simulink model "OMAP"  (R2018b)
settings: Solver=FixedStepDiscrete  StartTime=0.0  StopTime=10.0  FixedStep=0.01  RelTol=1e-3
values from neighbouring files (symbols this model uses):
  Clb_ICADirect_LaneDisp_StateFive = Simulink.Parameter    [omap_ver_442.m]
  Clb_ICADirect_LaneDisp_StateFour = Simulink.Parameter    [omap_ver_442.m]
  Clb_ICADirect_LaneDisp_StateOne = Simulink.Parameter    [omap_ver_442.m]
  Clb_ICADirect_LaneDisp_StateThree = Simulink.Parameter    [omap_ver_442.m]
  Clb_ICADirect_LaneDisp_StateTwo = Simulink.Parameter    [omap_ver_442.m]
  Clb_ICADirect_LaneDisp_StateZero = Simulink.Parameter    [omap_ver_442.m]
  Clb_ICADirect_LaneDispSW = Simulink.Parameter    [omap_ver_442.m]
  Clb_ICADirect_TrnLghtsCom_Switch = Simulink.Parameter    [omap_ver_442.m]
  Clb_ICADirect_TrnLghtsCom_Value = Simulink.Parameter    [omap_ver_442.m]
  Clb_ICADirect_TrnLghtsCrtl_Inhb = Simulink.Parameter    [omap_ver_442.m]
  OMAP_ACCAEB_EMSESC_Decel = Simulink.Parameter    [omap_ver_442.m]
  OMAP_ACCFCW_IC_Decel = Simulink.Parameter    [omap_ver_442.m]
  OMAP_clb_ACC_RVVReqType = Simulink.Parameter    [omap_ver_442.m]
  OMAP_clb_ACC_RVVReqType_Switch = Simulink.Parameter    [omap_ver_442.m]
  OMAP_clb_ACCHeadwayDisplay = Simulink.Parameter    [omap_ver_442.m]
  OMAP_clb_ACCHeadwayDisplay_Switch = Simulink.Parameter    [omap_ver_442.m]
  OMAP_clb_ACCHeadwayIcon = Simulink.Parameter    [omap_ver_442.m]
  OMAP_clb_ACCHeadwayIcon_Switch = Simulink.Parameter    [omap_ver_442.m]
  OMAP_clb_ACCMessagePrompt = Simulink.Parameter    [omap_ver_442.m]
  OMAP_clb_ACCMessagePrompt_Switch = Simulink.Parameter    [omap_ver_442.m]
  OMAP_clb_ACCRequestEPB = Simulink.Parameter    [omap_ver_442.m]
  OMAP_clb_ACCRequestEPB_Switch = Simulink.Parameter    [omap_ver_442.m]
  OMAP_clb_ACCSetSpeed = Simulink.Parameter    [omap_ver_442.m]
  OMAP_clb_ACCSetSpeed_Switch = Simulink.Parameter    [omap_ver_442.m]
  OMAP_clb_ACCSetSpeedDis = Simulink.Parameter    [omap_ver_442.m]
  OMAP_clb_ACCSetSpeedDis_Switch = Simulink.Parameter    [omap_ver_442.m]
  OMAP_clb_ACCState = Simulink.Parameter    [omap_ver_442.m]
  OMAP_clb_ACCState_Switch = Simulink.Parameter    [omap_ver_442.m]
  OMAP_clb_ACCStatusIconDis = Simulink.Parameter    [omap_ver_442.m]
  OMAP_clb_ACCStatusIconDis_Switch = Simulink.Parameter    [omap_ver_442.m]
  OMAP_clb_ACCTorqueReq = Simulink.Parameter    [omap_ver_442.m]
  OMAP_clb_ACCTorqueReq_Switch = Simulink.Parameter    [omap_ver_442.m]
  OMAP_clb_ADAS_State = Simulink.Parameter    [omap_ver_442.m]
  OMAP_clb_ADAS_State_Switch = Simulink.Parameter    [omap_ver_442.m]
  OMAP_clb_AEBAlertReq = Simulink.Parameter    [omap_ver_442.m]
  OMAP_clb_AEBAlertReq_Switch = Simulink.Parameter    [omap_ver_442.m]
  OMAP_clb_AEBBrakingProg = Simulink.Parameter    [omap_ver_442.m]
  OMAP_clb_AEBBrakingProg_Switch = Simulink.Parameter    [omap_ver_442.m]
  OMAP_clb_AEBFaultStatus = Simulink.Parameter    [omap_ver_442.m]
  OMAP_clb_AEBFaultStatus_Switch = Simulink.Parameter    [omap_ver_442.m]
  OMAP_clb_AEBMassageDisp = Simulink.Parameter    [omap_ver_442.m]
  OMAP_clb_AEBMassageDisp_Switch = Simulink.Parameter    [omap_ver_442.m]
  OMAP_clb_AEBState = Simulink.Parameter    [omap_ver_442.m]
  OMAP_clb_AEBState_Switch = Simulink.Parameter    [omap_ver_442.m]
  OMAP_clb_AEBSwitchStatus = Simulink.Parameter    [omap_ver_442.m]
  OMAP_clb_AEBSwitchStatus_Switch = Simulink.Parameter    [omap_ver_442.m]
  OMAP_clb_BrakeRequest = Simulink.Parameter    [omap_ver_442.m]
  OMAP_clb_BrakeRequest_Switch = Simulink.Parameter    [omap_ver_442.m]
  OMAP_clb_DecelerationSet = Simulink.Parameter    [omap_ver_442.m]
  OMAP_clb_DecelerationSet_Switch = Simulink.Parameter    [omap_ver_442.m]
  OMAP_clb_DecelerationType = Simulink.Parameter    [omap_ver_442.m]
  OMAP_clb_DecelerationType_Switch = Simulink.Parameter    [omap_ver_442.m]
  OMAP_clb_DeclControlReq = Simulink.Parameter    [omap_ver_442.m]
  OMAP_clb_DeclControlReq_Switch = Simulink.Parameter    [omap_ver_442.m]
  OMAP_clb_DownorUpGearMinTime = Simulink.Parameter    [omap_ver_442.m]
  OMAP_clb_DownorUpGearMinTime_Switch = Simulink.Parameter    [omap_ver_442.m]
  OMAP_clb_ELKPopupMessage = Simulink.Parameter    [omap_ver_442.m]
  OMAP_clb_ELKPopupMessage_Switch = Simulink.Parameter    [omap_ver_442.m]
  OMAP_clb_ELKSts = Simulink.Parameter    [omap_ver_442.m]
  OMAP_clb_ELKSts_Switch = Simulink.Parameter    [omap_ver_442.m]
  OMAP_clb_ESAFaultSt = Simulink.Parameter    [omap_ver_442.m]
  OMAP_clb_ESAFaultSt_Switch = Simulink.Parameter    [omap_ver_442.m]
  OMAP_clb_ESARequest = Simulink.Parameter    [omap_ver_442.m]
  OMAP_clb_ESARequest_Switch = Simulink.Parameter    [omap_ver_442.m]
  OMAP_clb_ESAState = Simulink.Parameter    [omap_ver_442.m]
  OMAP_clb_ESAState_Switch = Simulink.Parameter    [omap_ver_442.m]
  OMAP_clb_ESATorqueReq = Simulink.Parameter    [omap_ver_442.m]
  OMAP_clb_ESATorqueReq_Switch = Simulink.Parameter    [omap_ver_442.m]
  OMAP_clb_ESCDriveOff = Simulink.Parameter    [omap_ver_442.m]
  OMAP_clb_ESCDriveOff_Switch = Simulink.Parameter    [omap_ver_442.m]
  OMAP_clb_ESCHoldReq = Simulink.Parameter    [omap_ver_442.m]
  OMAP_clb_ESCHoldReq_Switch = Simulink.Parameter    [omap_ver_442.m]
  OMAP_clb_Handsoffwarning = Simulink.Parameter    [omap_ver_442.m]
  OMAP_clb_Handsoffwarning_Switch = Simulink.Parameter    [omap_ver_442.m]
  OMAP_clb_HapticAlarmReq = Simulink.Parameter    [omap_ver_442.m]
  OMAP_clb_HapticAlarmReq_Switch = Simulink.Parameter    [omap_ver_442.m]
  OMAP_clb_HMIPopupMassage = Simulink.Parameter    [omap_ver_442.m]
  OMAP_clb_HMIPopupMassage_Switch = Simulink.Parameter    [omap_ver_442.m]
  OMAP_clb_HWAActionSts = Simulink.Parameter    [omap_ver_442.m]
  OMAP_clb_HWAActionSts_Switch = Simulink.Parameter    [omap_ver_442.m]
  OMAP_clb_HWAMode = Simulink.Parameter    [omap_ver_442.m]
  OMAP_clb_HWAMode_Switch = Simulink.Parameter    [omap_ver_442.m]
  OMAP_clb_HWATurnOnIdctr = Simulink.Parameter    [omap_ver_442.m]
  OMAP_clb_HWATurnOnIdctr_Switch = Simulink.Parameter    [omap_ver_442.m]
  OMAP_clb_ICAMassageDisp = Simulink.Parameter    [omap_ver_442.m]
  OMAP_clb_ICAMassageDisp_Switch = Simulink.Parameter    [omap_ver_442.m]
  OMAP_clb_ICAStatusIcon = Simulink.Parameter    [omap_ver_442.m]
  OMAP_clb_ICAStatusIcon_Switch = Simulink.Parameter    [omap_ver_442.m]
  OMAP_clb_ISLCDriverRemind = Simulink.Parameter    [omap_ver_442.m]
  OMAP_clb_ISLCDriverRemind_Switch = Simulink.Parameter    [omap_ver_442.m]
  OMAP_clb_ISLCState = Simulink.Parameter    [omap_ver_442.m]
  OMAP_clb_ISLCState_Switch = Simulink.Parameter    [omap_ver_442.m]
  OMAP_clb_JAFaultSt = Simulink.Parameter    [omap_ver_442.m]
  OMAP_clb_JAFaultSt_Switch = Simulink.Parameter    [omap_ver_442.m]
  OMAP_clb_LCAPopupMessage = Simulink.Parameter    [omap_ver_442.m]
  OMAP_clb_LCAPopupMessage_Switch = Simulink.Parameter    [omap_ver_442.m]
  OMAP_clb_LCAStatusDisplay = Simulink.Parameter    [omap_ver_442.m]
  OMAP_clb_LCAStatusDisplay_Switch = Simulink.Parameter    [omap_ver_442.m]
  OMAP_clb_LDWStatusDisplay = Simulink.Parameter    [omap_ver_442.m]
  OMAP_clb_LDWStatusDisplay_Switch = Simulink.Parameter    [omap_ver_442.m]
  OMAP_clb_LDWWarningSt = Simulink.Parameter    [omap_ver_442.m]
  OMAP_clb_LDWWarningSt_Switch = Simulink.Parameter    [omap_ver_442.m]
  OMAP_clb_LightControlValid = Simulink.Parameter    [omap_ver_442.m]
  OMAP_clb_LightControlValid_Switch = Simulink.Parameter    [omap_ver_442.m]
  OMAP_clb_LKAActivation = Simulink.Parameter    [omap_ver_442.m]
  OMAP_clb_LKAActivation_Switch = Simulink.Parameter    [omap_ver_442.m]
  OMAP_clb_LKAAngleReq = Simulink.Parameter    [omap_ver_442.m]
  OMAP_clb_LKAAngleReq_Switch = Simulink.Parameter    [omap_ver_442.m]
  OMAP_clb_LKAMode = Simulink.Parameter    [omap_ver_442.m]
  OMAP_clb_LKAMode_Switch = Simulink.Parameter    [omap_ver_442.m]
  OMAP_clb_LKAorELK_CoolTime = Simulink.Parameter    [omap_ver_442.m]
  OMAP_clb_LKAState = Simulink.Parameter    [omap_ver_442.m]
  OMAP_clb_LKAState_Switch = Simulink.Parameter    [omap_ver_442.m]
  OMAP_clb_LKAStatusDisplay = Simulink.Parameter    [omap_ver_442.m]
  OMAP_clb_LKAStatusDisplay_Switch = Simulink.Parameter    [omap_ver_442.m]
  OMAP_clb_LKASwitchState = Simulink.Parameter    [omap_ver_442.m]
  OMAP_clb_LKASwitchState_Switch = Simulink.Parameter    [omap_ver_442.m]
  OMAP_clb_LKATorqFactReq = Simulink.Parameter    [omap_ver_442.m]
  OMAP_clb_LKATorqFactReq_Switch = Simulink.Parameter    [omap_ver_442.m]
  OMAP_clb_PrefillRequest = Simulink.Parameter    [omap_ver_442.m]
  ... (+36 more)
libraries: simulink x184, canmsglib x2
(part 5 of 14)

== system OMAP/Runnable_OMAP_10ms_sys/OMAP_Module/Default_IC ==
  Bus Creator16 : BusCreator  Inputs=36
  Constant3 : Constant  Value=0  OutDataTypeStr=uint8
  Constant4 : Constant  Value=0  OutDataTypeStr=uint8
  OMAPve_y_ACC_DesiredHeadway_DisplayNum : Constant  Value=0  OutDataTypeStr=uint8
  OMAPve_y_ACC_DesiredHeadway_Icon_BasicNum : Constant  Value=0  OutDataTypeStr=uint8
  OMAPve_y_ACC_Desired_Set_SpeedNum : Constant  Value=0  OutDataTypeStr=uint8
  OMAPve_y_ACC_HMI_TgtDisp_FlagNum : Constant  Value=0  OutDataTypeStr=uint8
  OMAPve_y_ACC_Pop_Up_MessageNum : Constant  Value=0  OutDataTypeStr=uint8
  OMAPve_y_ACC_Set_Speed_DisplayNum : Constant  Value=0  OutDataTypeStr=uint8
  OMAPve_y_ACC_Vehicle_Icon_DisplayNum : Constant  Value=0  OutDataTypeStr=uint8
  OMAPve_y_ADAS_ELKStsNum1 : Constant  Value=0  OutDataTypeStr=uint8
  OMAPve_y_ADAS_HWAActionSts : Constant  Value=0  OutDataTypeStr=uint8
  OMAPve_y_ADAS_HWAMode : Constant  Value=0  OutDataTypeStr=uint8
  OMAPve_y_ADAS_HWATurnOnIndicator : Constant  Value=0  OutDataTypeStr=uint8
  OMAPve_y_ADAS_ISLCDriverRemind1 : Constant  Value=0  OutDataTypeStr=uint8
  OMAPve_y_ADAS_ISLCState1 : Constant  Value=0  OutDataTypeStr=uint8
  OMAPve_y_ADAS_JAFaultSt_2 : Constant  Value=0  OutDataTypeStr=uint8
  OMAPve_y_ADAS_LightControlValid : Constant  Value=0  OutDataTypeStr=uint8
  OMAPve_y_ADAS_TurnLightsCommand1 : Constant  Value=0  OutDataTypeStr=uint8
  OMAPve_y_AEB_Alert_ReqNum : Constant  Value=0  OutDataTypeStr=uint8
  OMAPve_y_AEB_Fault_StatusNum : Constant  Value=0  OutDataTypeStr=uint8
  OMAPve_y_AEB_Switch_StatusNum : Constant  Value=0  OutDataTypeStr=uint8
  OMAPve_y_AEB_tipsNum : Constant  Value=0  OutDataTypeStr=uint8
  OMAPve_y_HMI_Popup_StatusNum : Constant  Value=0  OutDataTypeStr=uint8
  OMAPve_y_Hands_off_warningNum : Constant  Value=0  OutDataTypeStr=uint8
  OMAPve_y_ICA_HMI_Txt_DispNum : Constant  Value=0  OutDataTypeStr=uint8
  OMAPve_y_LDW_FlagNum : Constant  Value=0  OutDataTypeStr=uint8
  OMAPve_y_LDW_Status_DisplayNum : Constant  Value=0  OutDataTypeStr=uint8
  OMAPve_y_LKA_Mode_from_CameraNum : Constant  Value=0  OutDataTypeStr=uint8
  OMAPve_y_LKA_Status_DisplayNum : Constant  Value=0  OutDataTypeStr=uint8
  OMAPve_y_LKA_Switch_StateNum : Constant  Value=0  OutDataTypeStr=uint8
  OMAPve_y_LKA_action_indicationNum : Constant  Value=0  OutDataTypeStr=uint8
  OMAPve_y_RVVACC_Vehiclespeed_request_typeNum : Constant  Value=0  OutDataTypeStr=uint8
  OMAPve_y_TARGET_POSITIONNum : Constant  Value=0  OutDataTypeStr=uint8
  OMAPve_y_TJA_status_iconNum : Constant  Value=0  OutDataTypeStr=uint8
  OMAPve_y_TSR_Vision_Only_Sign_TypeNum : Constant  Value=0  OutDataTypeStr=uint8
  OMAPve_y_Vehicle_Lane_DisplayNum : Constant  Value=0  OutDataTypeStr=uint8
  Default_IC : Outport
  wires:
  OMAPve_y_LKA_Status_DisplayNum/1 -> Bus Creator16/31  "OMAPve_y_LKA_Status_Display_2"
  OMAPve_y_ACC_Desired_Set_SpeedNum/1 -> Bus Creator16/11  "OMAPve_y_ACC_Desired_Set_Speed_2"
  OMAPve_y_AEB_tipsNum/1 -> Bus Creator16/19  "OMAPve_y_AEB_tips_2"
  OMAPve_y_ACC_Pop_Up_MessageNum/1 -> Bus Creator16/15  "OMAPve_y_ACC_Pop_Up_Message_2"
  OMAPve_y_LDW_Status_DisplayNum/1 -> Bus Creator16/29  "OMAPve_y_LDW_Status_Display_2"
  OMAPve_y_AEB_Switch_StatusNum/1 -> Bus Creator16/18  "OMAPve_y_AEB_Switch_Status_2"
  OMAPve_y_ACC_DesiredHeadway_Icon_BasicNum/1 -> Bus Creator16/10  "OMAPve_y_ACC_DesiredHeadway_Icon_Basic_2"
  OMAPve_y_ICA_HMI_Txt_DispNum/1 -> Bus Creator16/35  "OMAPve_y_ICA_HMI_Txt_Disp_2"
  OMAPve_y_TARGET_POSITIONNum/1 -> Bus Creator16/22  "OMAPve_y_TARGET_POSITION_2"
  OMAPve_y_ACC_Vehicle_Icon_DisplayNum/1 -> Bus Creator16/13  "OMAPve_y_ACC_Vehicle_Icon_Display_2"
  OMAPve_y_ACC_DesiredHeadway_DisplayNum/1 -> Bus Creator16/9  "OMAPve_y_ACC_DesiredHeadway_Display_2"
  OMAPve_y_AEB_Alert_ReqNum/1 -> Bus Creator16/16  "OMAPve_y_AEB_Alert_Req_2"
  OMAPve_y_ACC_Set_Speed_DisplayNum/1 -> Bus Creator16/12  "OMAPve_y_ACC_Set_Speed_Display_2"
  OMAPve_y_LKA_action_indicationNum/1 -> Bus Creator16/33  "OMAPve_y_LKA_action_indication_2"
  OMAPve_y_Hands_off_warningNum/1 -> Bus Creator16/25  "OMAPve_y_Hands_off_warning_2"
  OMAPve_y_RVVACC_Vehiclespeed_request_typeNum/1 -> Bus Creator16/14  "OMAPve_y_RVVACC_Vehiclespeed_request_type_2"
  OMAPve_y_LKA_Mode_from_CameraNum/1 -> Bus Creator16/30  "OMAPve_y_LKA_Mode_from_Camera_2"
  OMAPve_y_ACC_HMI_TgtDisp_FlagNum/1 -> Bus Creator16/21  "OMAPve_y_ACC_HMI_TgtDisp_Flag_2"
  OMAPve_y_HMI_Popup_StatusNum/1 -> Bus Creator16/26  "OMAPve_y_HMI_Popup_Status_2"
  OMAPve_y_TSR_Vision_Only_Sign_TypeNum/1 -> Bus Creator16/8  "OMAPve_y_TSR_Vision_Only_Sign_Type_2"
  OMAPve_y_TJA_status_iconNum/1 -> Bus Creator16/36  "OMAPve_y_TJA_status_icon_2"
  OMAPve_y_AEB_Fault_StatusNum/1 -> Bus Creator16/17  "OMAPve_y_AEB_Fault_Status_2"
  OMAPve_y_Vehicle_Lane_DisplayNum/1 -> Bus Creator16/27  "OMAPve_y_Vehicle_Lane_Display_2"
  OMAPve_y_LKA_Switch_StateNum/1 -> Bus Creator16/32  "OMAPve_y_LKA_Switch_State_2"
  OMAPve_y_LDW_FlagNum/1 -> Bus Creator16/28  "OMAPve_y_LDW_Flag_2"
  Bus Creator16/1 -> Default_IC/1  "Default_IC"
  OMAPve_y_ADAS_ELKStsNum1/1 -> Bus Creator16/34  "OMAPve_y_ADAS_ELKSts_2"
  OMAPve_y_ADAS_JAFaultSt_2/1 -> Bus Creator16/20  "OMAPve_y_ADAS_JAFaultSt_2"
  OMAPve_y_ADAS_ISLCState1/1 -> Bus Creator16/23  "OMAPve_y_ADAS_ISLCState_2"
  OMAPve_y_ADAS_ISLCDriverRemind1/1 -> Bus Creator16/24  "OMAPve_y_ADAS_ISLCDriverRemind_2"
  OMAPve_y_ADAS_LightControlValid/1 -> Bus Creator16/6  "OMAPve_y_ADAS_LightControlValid_2"
  OMAPve_y_ADAS_HWAActionSts/1 -> Bus Creator16/4  "OMAPve_y_ADAS_HWAActionSts_2"
  OMAPve_y_ADAS_HWATurnOnIndicator/1 -> Bus Creator16/3  "OMAPve_y_ADAS_HWATurnOnIndicator_2"
  OMAPve_y_ADAS_HWAMode/1 -> Bus Creator16/7  "OMAPve_y_ADAS_HWAMode_2"
  OMAPve_y_ADAS_TurnLightsCommand1/1 -> Bus Creator16/5  "OMAPve_y_ADAS_TurnLightsCommand_2"
  Constant3/1 -> Bus Creator16/2  "OMAPve_y_ADAS_ESAFaultSt_2"
  Constant4/1 -> Bus Creator16/1  "OMAPve_y_ADAS_ELKPopupMessage_2"

== system OMAP/Runnable_OMAP_10ms_sys/OMAP_Module/Default_OTHER ==
  Bus Creator26 : BusCreator  Inputs=5
  Data Type Conversion72 : DataTypeConversion  OutDataTypeStr=uint8
  Delay : Delay
  NOT : Logic  Operator=NOT  IconShape=distinctive  AllPortsSameDT=off  OutDataTypeStr=boolean
  OMAPve_y_ABS_ESP_power_cut_request2Num1 : Constant  Value=0  OutDataTypeStr=uint8
  OMAPve_y_ASR_connection_dis_demand2Num1 : Constant  Value=0  OutDataTypeStr=uint8
  OMAPve_y_ECU_operating_phaseNum1 : Constant  Value=9  OutDataTypeStr=uint8
  OMAPve_y_Radar_StateNum1 : Constant  Value=2  OutDataTypeStr=uint8
  Default : Outport
  wires:
  OMAPve_y_ASR_connection_dis_demand2Num1/1 -> Bus Creator26/2  "OMAPve_y_ASR_connection_dis_demand2_2"
  OMAPve_y_ABS_ESP_power_cut_request2Num1/1 -> Bus Creator26/1  "OMAPve_y_ABS_ESP_power_cut_request2_2"
  Data Type Conversion72/1 -> Bus Creator26/3  "OMAPve_y_TYPE_RAPPORT_2"
  Bus Creator26/1 -> Default/1  "Default"
  OMAPve_y_Radar_StateNum1/1 -> Bus Creator26/5  "OMAPve_y_Radar_State_2"
  OMAPve_y_ECU_operating_phaseNum1/1 -> Bus Creator26/4  "OMAPve_y_ECU_operating_phase_2"
  NOT/1 -> Delay/1, Data Type Conversion72/1
  Delay/1 -> NOT/1

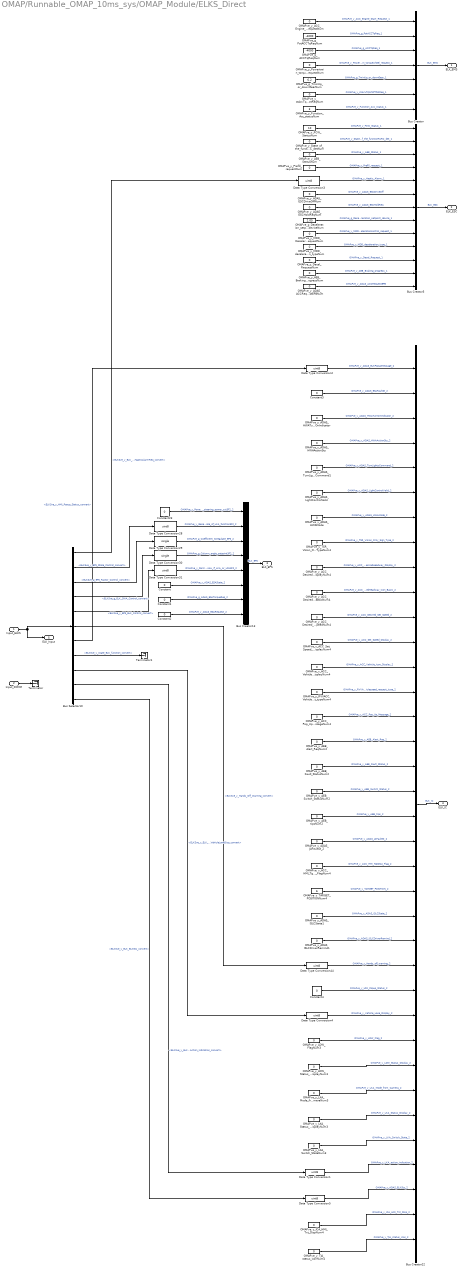
== system OMAP/Runnable_OMAP_10ms_sys/OMAP_Module/ELKS_Direct ==
  Input_ELKS : Inport
  Input_FDMM : Inport  Port=2
  Bus Creator : BusCreator  Inputs=7
  Bus Creator13 : BusCreator  Inputs=8
  Bus Creator22 : BusCreator  Inputs=36
  Bus Creator5 : BusCreator  Inputs=13
  Bus Selector10 : BusSelector  OutputSignals=ELKSve_y_ELK_HapticAlarmReq_convert,ELKSve_y_EPS_State_Control_convert,ELKSve_g_EPS_Factor_Control_convert,ELKSve_g_ELK_SWA_Control_convert,ELKSve_y_EPS_ELK_Control_convert,ELKSve_y_Hands_Off_Warning_convert,ELKSve_y_HMI_Popup_Status_convert,ELKSve_y_state_ELK_function_convert,ELKSve_y_ELK_VehicleLaneDisp_convert,ELKSve_y_ELK_Action_Indication_convert,ELKSve_y_ELK_ELKSts_convert
  Constant{,2..4,23} (5 alike) : Constant  Value=0  OutDataTypeStr=uint8
  Constant1 : Constant  Value=0  OutDataTypeStr=single
  Data Type Conversion{1..5,28,31,44} (8 alike) : DataTypeConversion  OutDataTypeStr=uint8
  Data Type Conversion29 : DataTypeConversion  OutDataTypeStr=single
  Data Type Conversion30 : DataTypeConversion  OutDataTypeStr=single
  OMAPve_g_ACCTqReqNum : Constant  Value=-4000  OutDataTypeStr=single
  OMAPve_g_Deceleration_setpoint_deviceNum : Constant  Value=2.05  OutDataTypeStr=single
  OMAPve_g_PotACCTqReqNum : Constant  Value=-4000  OutDataTypeStr=single
  OMAPve_g_TminUp_or_downGearNum : Constant  Value=6.2  OutDataTypeStr=single
  OMAPve_y_ACC_DesiredHeadway_DisplayNum4 : Constant  Value=0  OutDataTypeStr=uint8
  OMAPve_y_ACC_DesiredHeadway_Icon_BasicNum4 : Constant  Value=0  OutDataTypeStr=uint8
  OMAPve_y_ACC_Desired_Set_SpeedNum4 : Constant  Value=0  OutDataTypeStr=uint8
  OMAPve_y_ACC_Engine_Start_RequestNum : Constant  Value=0  OutDataTypeStr=uint8
  OMAPve_y_ACC_HMI_TgtDisp_FlagNum4 : Constant  Value=0  OutDataTypeStr=uint8
  OMAPve_y_ACC_Pop_Up_MessageNum4 : Constant  Value=0  OutDataTypeStr=uint8
  OMAPve_y_ACC_Set_Speed_DisplayNum4 : Constant  Value=0  OutDataTypeStr=uint8
  OMAPve_y_ACC_Vehicle_Icon_DisplayNum4 : Constant  Value=0  OutDataTypeStr=uint8
  OMAPve_y_ADAS_ACCRequestEPBNum : Constant  Value=0  OutDataTypeStr=uint8
  OMAPve_y_ADAS_ESCDriveOffNum : Constant  Value=0  OutDataTypeStr=uint8
  OMAPve_y_ADAS_ESCHoldReqNum : Constant  Value=0  OutDataTypeStr=uint8
  OMAPve_y_ADAS_HWAActionSts : Constant  Value=0  OutDataTypeStr=uint8
  OMAPve_y_ADAS_HWAMode : Constant  Value=0  OutDataTypeStr=uint8
  OMAPve_y_ADAS_HWATurnOnIndicator : Constant  Value=0  OutDataTypeStr=uint8
  OMAPve_y_ADAS_ISLCDriverRemind1 : Constant  Value=0  OutDataTypeStr=uint8
  OMAPve_y_ADAS_ISLCState1 : Constant  Value=0  OutDataTypeStr=uint8
  OMAPve_y_ADAS_JAFaultSt_2 : Constant  Value=0  OutDataTypeStr=uint8
  OMAPve_y_ADAS_LightControlValid : Constant  Value=0  OutDataTypeStr=uint8
  OMAPve_y_ADAS_TurnLightsCommand1 : Constant  Value=0  OutDataTypeStr=uint8
  OMAPve_y_AEB_Alert_ReqNum2 : Constant  Value=0  OutDataTypeStr=uint8
  OMAPve_y_AEB_Braking_progressNum : Constant  Value=0  OutDataTypeStr=uint8
  OMAPve_y_AEB_Fault_StatusNum2 : Constant  Value=0  OutDataTypeStr=uint8
  OMAPve_y_AEB_StatusNum : Constant  Value=0  OutDataTypeStr=uint8
  OMAPve_y_AEB_Switch_StatusNum2 : Constant  Value=0  OutDataTypeStr=uint8
  OMAPve_y_AEB_tipsNum2 : Constant  Value=0  OutDataTypeStr=uint8
  OMAPve_y_Decel_RequestNum : Constant  Value=0  OutDataTypeStr=uint8
  OMAPve_y_FCW_StatusNum : Constant  Value=10  OutDataTypeStr=uint8
  OMAPve_y_Function_Acc_statusNum : Constant  Value=3  OutDataTypeStr=uint8
  OMAPve_y_ICA_HMI_Txt_DispNum4 : Constant  Value=0  OutDataTypeStr=uint8
  OMAPve_y_LDW_FlagNum3 : Constant  Value=0  OutDataTypeStr=uint8
  OMAPve_y_LDW_Status_DisplayNum3 : Constant  Value=0  OutDataTypeStr=uint8
  OMAPve_y_LKA_Mode_from_CameraNum3 : Constant  Value=0  OutDataTypeStr=uint8
  OMAPve_y_LKA_Status_DisplayNum3 : Constant  Value=0  OutDataTypeStr=uint8
  OMAPve_y_LKA_Switch_StateNum3 : Constant  Value=0  OutDataTypeStr=uint8
  OMAPve_y_MDD_Decelerationcontrol_requestNum : Constant  Value=0  OutDataTypeStr=uint8
  OMAPve_y_MDD_deceleration_typeNum : Constant  Value=0  OutDataTypeStr=uint8
  OMAPve_y_Powertrain_torquewheel_requestNum : Constant  Value=0  OutDataTypeStr=uint8
  OMAPve_y_Prefill_requestNum : Constant  Value=0  OutDataTypeStr=uint8
  OMAPve_y_RVVACC_Vehiclespeed_request_typeNum4 : Constant  Value=0  OutDataTypeStr=uint8
  OMAPve_y_State_of_the_functionFARC_detNum : Constant  Value=0  OutDataTypeStr=uint8
  OMAPve_y_TARGET_POSITIONNum4 : Constant  Value=6  OutDataTypeStr=uint8
  OMAPve_y_TJA_status_iconNum4 : Constant  Value=0  OutDataTypeStr=uint8
  OMAPve_y_TSR_Vision_Only_Sign_TypeNum4 : Constant  Value=0  OutDataTypeStr=uint8
  OMAPve_y_stAcvTqWhlPTPotReqNum : Constant  Value=0  OutDataTypeStr=uint8
  Terminator : Terminator
  Terminator1 : Terminator
  ELK_EMS : Outport
  ELK_ESC : Outport  Port=2
  ELK_EPS : Outport  Port=3
  ELK_IC : Outport  Port=4
  ELK_Input : Outport  Port=5
  wires:
  Bus Creator22/1 -> ELK_IC/1  "ELK_IC"
  Data Type Conversion44/1 -> Bus Creator22/25  "OMAPve_y_Hands_off_warning_2"
  Data Type Conversion1/1 -> Bus Creator22/33  "OMAPve_y_LKA_action_indication_2"
  Bus Selector10/5 -> Data Type Conversion31/1  "<ELKSve_y_EPS_ELK_Control_convert>"
  Bus Selector10/2 -> Data Type Conversion28/1  "<ELKSve_y_EPS_State_Control_convert>"
  Data Type Conversion29/1 -> Bus Creator13/3  "OMAPve_g_Coefficient_toregulate_EPS_2"
  OMAPve_y_LDW_Status_DisplayNum3/1 -> Bus Creator22/29  "OMAPve_y_LDW_Status_Display_2"
  OMAPve_y_LDW_FlagNum3/1 -> Bus Creator22/28  "OMAPve_y_LDW_Flag_2"
  OMAPve_y_ACC_DesiredHeadway_Icon_BasicNum4/1 -> Bus Creator22/10  "OMAPve_y_ACC_DesiredHeadway_Icon_Basic_2"
  Bus Selector10/6 -> Data Type Conversion44/1  "<ELKSve_y_Hands_Off_Warning_convert>"
  Bus Selector10/4 -> Data Type Conversion30/1  "<ELKSve_g_ELK_SWA_Control_convert>"
  OMAPve_y_ACC_HMI_TgtDisp_FlagNum4/1 -> Bus Creator22/21  "OMAPve_y_ACC_HMI_TgtDisp_Flag_2"
  Bus Selector10/3 -> Data Type Conversion29/1  "<ELKSve_g_EPS_Factor_Control_convert>"
  Data Type Conversion4/1 -> Bus Creator22/27  "OMAPve_y_Vehicle_Lane_Display_2"
  OMAPve_y_TJA_status_iconNum4/1 -> Bus Creator22/36  "OMAPve_y_TJA_status_icon_2"
  Bus Selector10/8 -> Terminator1/1  "<ELKSve_y_state_ELK_function_convert>"
  OMAPve_y_TARGET_POSITIONNum4/1 -> Bus Creator22/22  "OMAPve_y_TARGET_POSITION_2"
  OMAPve_y_ACC_Vehicle_Icon_DisplayNum4/1 -> Bus Creator22/13  "OMAPve_y_ACC_Vehicle_Icon_Display_2"
  OMAPve_y_ACC_DesiredHeadway_DisplayNum4/1 -> Bus Creator22/9  "OMAPve_y_ACC_DesiredHeadway_Display_2"
  OMAPve_y_LKA_Status_DisplayNum3/1 -> Bus Creator22/31  "OMAPve_y_LKA_Status_Display_2"
  OMAPve_y_AEB_tipsNum2/1 -> Bus Creator22/19  "OMAPve_y_AEB_tips_2"
  OMAPve_y_ACC_Pop_Up_MessageNum4/1 -> Bus Creator22/15  "OMAPve_y_ACC_Pop_Up_Message_2"
  Bus Selector10/7 -> Data Type Conversion2/1  "<ELKSve_y_HMI_Popup_Status_convert>"
  OMAPve_y_ACC_Desired_Set_SpeedNum4/1 -> Bus Creator22/11  "OMAPve_y_ACC_Desired_Set_Speed_2"
  OMAPve_y_ICA_HMI_Txt_DispNum4/1 -> Bus Creator22/35  "OMAPve_y_ICA_HMI_Txt_Disp_2"
  Bus Creator13/1 -> ELK_EPS/1  "ELK_EPS"
  OMAPve_y_AEB_Fault_StatusNum2/1 -> Bus Creator22/17  "OMAPve_y_AEB_Fault_Status_2"
  Constant4/1 -> Bus Creator22/26  "OMAPve_y_HMI_Popup_Status_2"
  OMAPve_y_AEB_Switch_StatusNum2/1 -> Bus Creator22/18  "OMAPve_y_AEB_Switch_Status_2"
  OMAPve_y_LKA_Mode_from_CameraNum3/1 -> Bus Creator22/30  "OMAPve_y_LKA_Mode_from_Camera_2"
  OMAPve_y_AEB_Alert_ReqNum2/1 -> Bus Creator22/16  "OMAPve_y_AEB_Alert_Req_2"
  OMAPve_y_ACC_Set_Speed_DisplayNum4/1 -> Bus Creator22/12  "OMAPve_y_ACC_Set_Speed_Display_2"
  Input_ELKS/1 -> ELK_Input/1, Bus Selector10/1
  Constant23/1 -> Bus Creator13/1  "OMAPve_y_Power_steering_power_cut3F2_2"
  Data Type Conversion30/1 -> Bus Creator13/4  "OMAPve_g_Column_angle_setpoint3F2_2"
  OMAPve_y_LKA_Switch_StateNum3/1 -> Bus Creator22/32  "OMAPve_y_LKA_Switch_State_2"
  Data Type Conversion28/1 -> Bus Creator13/2  "OMAPve_y_General_state_of_LKA_function3F2_2"
  Data Type Conversion31/1 -> Bus Creator13/5  "OMAPve_y_Permit_to_know_if_LKA_or_LPA3F2_2"
  OMAPve_y_RVVACC_Vehiclespeed_request_typeNum4/1 -> Bus Creator22/14  "OMAPve_y_RVVACC_Vehiclespeed_request_type_2"
  OMAPve_y_TSR_Vision_Only_Sign_TypeNum4/1 -> Bus Creator22/8  "OMAPve_y_TSR_Vision_Only_Sign_Type_2"
  OMAPve_y_Function_Acc_statusNum/1 -> Bus Creator/7  "OMAPve_y_Function_Acc_status_1"
  OMAPve_y_stAcvTqWhlPTPotReqNum/1 -> Bus Creator/6  "OMAPve_y_stAcvTqWhlPTPotReq_1"
  Bus Creator/1 -> ELK_EMS/1  "ELK_EMS"
  OMAPve_y_ACC_Engine_Start_RequestNum/1 -> Bus Creator/1  "OMAPve_y_ACC_Engine_Start_Request_1"
  OMAPve_g_TminUp_or_downGearNum/1 -> Bus Creator/5  "OMAPve_g_TminUp_or_downGear_1"
  OMAPve_g_PotACCTqReqNum/1 -> Bus Creator/2  "OMAPve_g_PotACCTqReq_1"
  OMAPve_y_Powertrain_torquewheel_requestNum/1 -> Bus Creator/4  "OMAPve_y_Powertrain_torquewheel_request_1"
  OMAPve_g_ACCTqReqNum/1 -> Bus Creator/3  "OMAPve_g_ACCTqReq_1"
  OMAPve_g_Deceleration_setpoint_deviceNum/1 -> Bus Creator5/8  "OMAPve_g_Deceleration_setpoint_device_1"
  OMAPve_y_AEB_StatusNum/1 -> Bus Creator5/3  "OMAPve_y_AEB_Status_1"
  Data Type Conversion3/1 -> Bus Creator5/5  "OMAPve_y_Haptic_Alarm_1"
  OMAPve_y_AEB_Braking_progressNum/1 -> Bus Creator5/12  "OMAPve_y_AEB_Braking_progress_1"
  OMAPve_y_FCW_StatusNum/1 -> Bus Creator5/1  "OMAPve_y_FCW_Status_1"
  OMAPve_y_Decel_RequestNum/1 -> Bus Creator5/11  "OMAPve_y_Decel_Request_1"
  OMAPve_y_MDD_Decelerationcontrol_requestNum/1 -> Bus Creator5/9  "OMAPve_y_MDD_Decelerationcontrol_request_1"
  OMAPve_y_MDD_deceleration_typeNum/1 -> Bus Creator5/10  "OMAPve_y_MDD_deceleration_type_1"
  OMAPve_y_State_of_the_functionFARC_detNum/1 -> Bus Creator5/2  "OMAPve_y_State_of_the_functionFARC_det_1"
  OMAPve_y_Prefill_requestNum/1 -> Bus Creator5/4  "OMAPve_y_Prefill_request_1"
  Bus Creator5/1 -> ELK_ESC/1  "ELK_ESC"
  Input_FDMM/1 -> Terminator/1
  Bus Selector10/10 -> Data Type Conversion1/1  "<ELKSve_y_ELK_Action_Indication_convert>"
  Bus Selector10/1 -> Data Type Conversion3/1  "<ELKSve_y_ELK_HapticAlarmReq_convert>"
  Bus Selector10/11 -> Data Type Conversion5/1  "<ELKSve_y_ELK_ELKSts_convert>"
  Bus Selector10/9 -> Data Type Conversion4/1  "<ELKSve_y_ELK_VehicleLaneDisp_convert>"
  Data Type Conversion5/1 -> Bus Creator22/34  "OMAPve_y_ADAS_ELKSts_2"
  OMAPve_y_ADAS_ESCHoldReqNum/1 -> Bus Creator5/7  "OMAPve_y_ADAS_ESCHoldReq"
  OMAPve_y_ADAS_ESCDriveOffNum/1 -> Bus Creator5/6  "OMAPve_y_ADAS_ESCDriveOff"
  OMAPve_y_ADAS_ACCRequestEPBNum/1 -> Bus Creator5/13  "OMAPve_y_ADAS_ACCRequestEPB"
  OMAPve_y_ADAS_JAFaultSt_2/1 -> Bus Creator22/20  "OMAPve_y_ADAS_JAFaultSt_2"
  OMAPve_y_ADAS_ISLCState1/1 -> Bus Creator22/23  "OMAPve_y_ADAS_ISLCState_2"
  OMAPve_y_ADAS_ISLCDriverRemind1/1 -> Bus Creator22/24  "OMAPve_y_ADAS_ISLCDriverRemind_2"
  OMAPve_y_ADAS_LightControlValid/1 -> Bus Creator22/6  "OMAPve_y_ADAS_LightControlValid_2"
  OMAPve_y_ADAS_HWAActionSts/1 -> Bus Creator22/4  "OMAPve_y_ADAS_HWAActionSts_2"
  OMAPve_y_ADAS_HWATurnOnIndicator/1 -> Bus Creator22/3  "OMAPve_y_ADAS_HWATurnOnIndicator_2"
  OMAPve_y_ADAS_HWAMode/1 -> Bus Creator22/7  "OMAPve_y_ADAS_HWAMode_2"
  OMAPve_y_ADAS_TurnLightsCommand1/1 -> Bus Creator22/5  "OMAPve_y_ADAS_TurnLightsCommand_2"
  Constant1/1 -> Bus Creator13/7  "OMAPve_g_ADAS_ESATorqueReq_2"
  Constant/1 -> Bus Creator13/6  "OMAPve_y_ADAS_ESAState_2"
  Constant2/1 -> Bus Creator13/8  "OMAPve_y_ADAS_ESARequest_2"
  Constant3/1 -> Bus Creator22/2  "OMAPve_y_ADAS_ESAFaultSt_2"
  Data Type Conversion2/1 -> Bus Creator22/1  "OMAPve_y_ADAS_ELKPopupMessage_2"

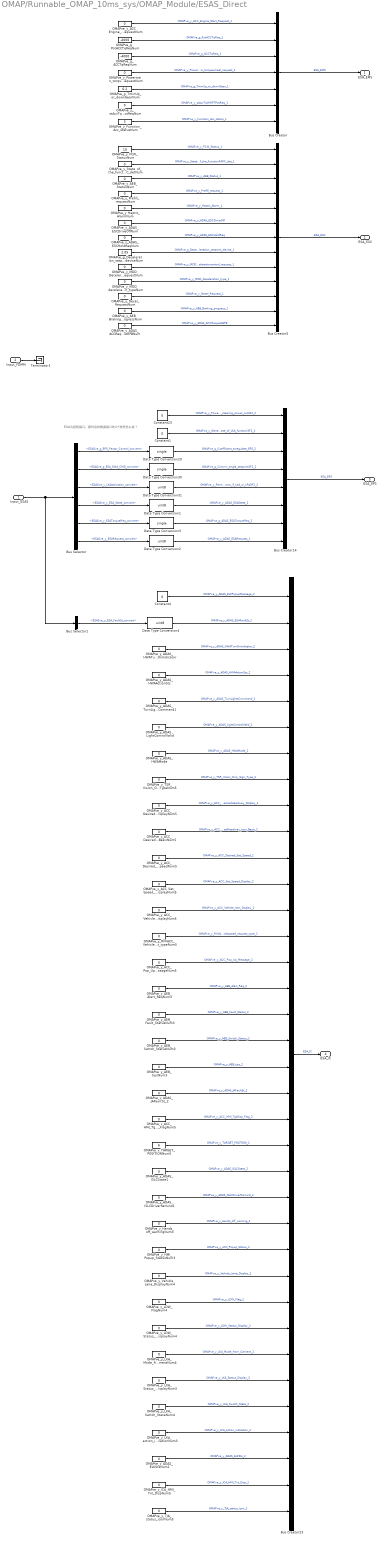
== system OMAP/Runnable_OMAP_10ms_sys/OMAP_Module/ESAS_Direct ==
  note: ESA为扭矩接口。那对应的角度接口的4个信号怎么发？
  Input_ESAS : Inport
  Input_FDMM : Inport  Port=2
  Bus Creator : BusCreator  Inputs=7
  Bus Creator14 : BusCreator  Inputs=8
  Bus Creator23 : BusCreator  Inputs=36
  Bus Creator5 : BusCreator  Inputs=13
  Bus Selector : BusSelector  OutputSignals=ESASve_g_EPS_Factor_Control_convert,ESASve_g_ESA_SWA_CMD_convert,ESASve_y_LKAActivation_convert,ESASve_y_ESA_State_convert,ESASve_y_ESATorqueReq_convert,ESASve_y_ESARequest_convert
  Bus Selector1 : BusSelector  OutputSignals=ESASve_y_ESA_FaultSt_convert
  Constant1 : Constant  Value=0  OutDataTypeStr=uint8
  Constant23 : Constant  Value=0  OutDataTypeStr=uint8
  Constant4 : Constant  Value=0  OutDataTypeStr=uint8
  Data Type Conversion{1..2,4,31} (4 alike) : DataTypeConversion  OutDataTypeStr=uint8
  Data Type Conversion29 : DataTypeConversion  OutDataTypeStr=single
  Data Type Conversion3 : DataTypeConversion  OutDataTypeStr=single
  Data Type Conversion30 : DataTypeConversion  OutDataTypeStr=single
  OMAPve_g_ACCTqReqNum : Constant  Value=-4000  OutDataTypeStr=single
  OMAPve_g_Deceleration_setpoint_deviceNum : Constant  Value=2.05  OutDataTypeStr=single
  OMAPve_g_PotACCTqReqNum : Constant  Value=-4000  OutDataTypeStr=single
  OMAPve_g_TminUp_or_downGearNum : Constant  Value=6.2  OutDataTypeStr=single
  OMAPve_y_ACC_DesiredHeadway_DisplayNum5 : Constant  Value=0  OutDataTypeStr=uint8
  OMAPve_y_ACC_DesiredHeadway_Icon_BasicNum5 : Constant  Value=0  OutDataTypeStr=uint8
  OMAPve_y_ACC_Desired_Set_SpeedNum5 : Constant  Value=0  OutDataTypeStr=uint8
  OMAPve_y_ACC_Engine_Start_RequestNum : Constant  Value=0  OutDataTypeStr=uint8
  OMAPve_y_ACC_HMI_TgtDisp_FlagNum5 : Constant  Value=0  OutDataTypeStr=uint8
  OMAPve_y_ACC_Pop_Up_MessageNum5 : Constant  Value=0  OutDataTypeStr=uint8
  OMAPve_y_ACC_Set_Speed_DisplayNum5 : Constant  Value=0  OutDataTypeStr=uint8
  OMAPve_y_ACC_Vehicle_Icon_DisplayNum5 : Constant  Value=0  OutDataTypeStr=uint8
  OMAPve_y_ADAS_ACCRequestEPBNum : Constant  Value=0  OutDataTypeStr=uint8
  OMAPve_y_ADAS_ELKStsNum1 : Constant  Value=0  OutDataTypeStr=uint8
  OMAPve_y_ADAS_ESCDriveOffNum : Constant  Value=0  OutDataTypeStr=uint8
  OMAPve_y_ADAS_ESCHoldReqNum : Constant  Value=0  OutDataTypeStr=uint8
  OMAPve_y_ADAS_HWAActionSts : Constant  Value=0  OutDataTypeStr=uint8
  OMAPve_y_ADAS_HWAMode : Constant  Value=0  OutDataTypeStr=uint8
  OMAPve_y_ADAS_HWATurnOnIndicator : Constant  Value=0  OutDataTypeStr=uint8
  OMAPve_y_ADAS_ISLCDriverRemind1 : Constant  Value=0  OutDataTypeStr=uint8
  OMAPve_y_ADAS_ISLCState1 : Constant  Value=0  OutDataTypeStr=uint8
  OMAPve_y_ADAS_JAFaultSt_2 : Constant  Value=0  OutDataTypeStr=uint8
  OMAPve_y_ADAS_LightControlValid : Constant  Value=0  OutDataTypeStr=uint8
  OMAPve_y_ADAS_TurnLightsCommand1 : Constant  Value=0  OutDataTypeStr=uint8
  OMAPve_y_AEB_Alert_ReqNum3 : Constant  Value=0  OutDataTypeStr=uint8
  OMAPve_y_AEB_Braking_progressNum : Constant  Value=0  OutDataTypeStr=uint8
  OMAPve_y_AEB_Fault_StatusNum3 : Constant  Value=0  OutDataTypeStr=uint8
  OMAPve_y_AEB_StatusNum : Constant  Value=0  OutDataTypeStr=uint8
  OMAPve_y_AEB_Switch_StatusNum3 : Constant  Value=0  OutDataTypeStr=uint8
  OMAPve_y_AEB_tipsNum3 : Constant  Value=0  OutDataTypeStr=uint8
  OMAPve_y_Decel_RequestNum : Constant  Value=0  OutDataTypeStr=uint8
  OMAPve_y_FCW_StatusNum : Constant  Value=10  OutDataTypeStr=uint8
  OMAPve_y_Function_Acc_statusNum : Constant  Value=3  OutDataTypeStr=uint8
  OMAPve_y_HMI_Popup_StatusNum3 : Constant  Value=0  OutDataTypeStr=uint8
  OMAPve_y_Hands_off_warningNum3 : Constant  Value=0  OutDataTypeStr=uint8
  OMAPve_y_Haptic_AlarmNum : Constant  Value=0  OutDataTypeStr=uint8
  OMAPve_y_ICA_HMI_Txt_DispNum5 : Constant  Value=0  OutDataTypeStr=uint8
  OMAPve_y_LDW_FlagNum4 : Constant  Value=0  OutDataTypeStr=uint8
  OMAPve_y_LDW_Status_DisplayNum4 : Constant  Value=0  OutDataTypeStr=uint8
  OMAPve_y_LKA_Mode_from_CameraNum4 : Constant  Value=0  OutDataTypeStr=uint8
  OMAPve_y_LKA_Status_DisplayNum3 : Constant  Value=0  OutDataTypeStr=uint8
  OMAPve_y_LKA_Switch_StateNum4 : Constant  Value=0  OutDataTypeStr=uint8
  OMAPve_y_LKA_action_indicationNum3 : Constant  Value=0  OutDataTypeStr=uint8
  OMAPve_y_MDD_Decelerationcontrol_requestNum : Constant  Value=0  OutDataTypeStr=uint8
  OMAPve_y_MDD_deceleration_typeNum : Constant  Value=0  OutDataTypeStr=uint8
  OMAPve_y_Powertrain_torquewheel_requestNum : Constant  Value=0  OutDataTypeStr=uint8
  OMAPve_y_Prefill_requestNum : Constant  Value=0  OutDataTypeStr=uint8
  OMAPve_y_RVVACC_Vehiclespeed_request_typeNum5 : Constant  Value=0  OutDataTypeStr=uint8
  OMAPve_y_State_of_the_functionFARC_detNum : Constant  Value=0  OutDataTypeStr=uint8
  OMAPve_y_TARGET_POSITIONNum5 : Constant  Value=6  OutDataTypeStr=uint8
  OMAPve_y_TJA_status_iconNum5 : Constant  Value=0  OutDataTypeStr=uint8
  OMAPve_y_TSR_Vision_Only_Sign_TypeNum5 : Constant  Value=0  OutDataTypeStr=uint8
  OMAPve_y_Vehicle_Lane_DisplayNum4 : Constant  Value=0  OutDataTypeStr=uint8
  OMAPve_y_stAcvTqWhlPTPotReqNum : Constant  Value=0  OutDataTypeStr=uint8
  Terminator1 : Terminator
  ESA_EMS : Outport
  ESA_ESC : Outport  Port=2
  ESA_EPS : Outport  Port=3
  ESA_IC : Outport  Port=4
  wires:
  Bus Creator23/1 -> ESA_IC/1  "ESA_IC"
  Bus Creator14/1 -> ESA_EPS/1  "ESA_EPS"
  OMAPve_y_AEB_Fault_StatusNum3/1 -> Bus Creator23/17  "OMAPve_y_AEB_Fault_Status_2"
  OMAPve_y_ACC_Vehicle_Icon_DisplayNum5/1 -> Bus Creator23/13  "OMAPve_y_ACC_Vehicle_Icon_Display_2"
  OMAPve_y_TSR_Vision_Only_Sign_TypeNum5/1 -> Bus Creator23/8  "OMAPve_y_TSR_Vision_Only_Sign_Type_2"
  OMAPve_y_AEB_Alert_ReqNum3/1 -> Bus Creator23/16  "OMAPve_y_AEB_Alert_Req_2"
  OMAPve_y_TJA_status_iconNum5/1 -> Bus Creator23/36  "OMAPve_y_TJA_status_icon_2"
  OMAPve_y_TARGET_POSITIONNum5/1 -> Bus Creator23/22  "OMAPve_y_TARGET_POSITION_2"
  OMAPve_y_AEB_Switch_StatusNum3/1 -> Bus Creator23/18  "OMAPve_y_AEB_Switch_Status_2"
  OMAPve_y_AEB_tipsNum3/1 -> Bus Creator23/19  "OMAPve_y_AEB_tips_2"
  OMAPve_y_ICA_HMI_Txt_DispNum5/1 -> Bus Creator23/35  "OMAPve_y_ICA_HMI_Txt_Disp_2"
  OMAPve_y_ACC_Desired_Set_SpeedNum5/1 -> Bus Creator23/11  "OMAPve_y_ACC_Desired_Set_Speed_2"
  OMAPve_y_ACC_DesiredHeadway_DisplayNum5/1 -> Bus Creator23/9  "OMAPve_y_ACC_DesiredHeadway_Display_2"
  OMAPve_y_LKA_Switch_StateNum4/1 -> Bus Creator23/32  "OMAPve_y_LKA_Switch_State_2"
  OMAPve_y_LKA_Status_DisplayNum3/1 -> Bus Creator23/31  "OMAPve_y_LKA_Status_Display_2"
  OMAPve_y_LDW_Status_DisplayNum4/1 -> Bus Creator23/29  "OMAPve_y_LDW_Status_Display_2"
  OMAPve_y_ACC_Pop_Up_MessageNum5/1 -> Bus Creator23/15  "OMAPve_y_ACC_Pop_Up_Message_2"
  OMAPve_y_ACC_Set_Speed_DisplayNum5/1 -> Bus Creator23/12  "OMAPve_y_ACC_Set_Speed_Display_2"
  Data Type Conversion30/1 -> Bus Creator14/4  "OMAPve_g_Column_angle_setpoint3F2_2"
  OMAPve_y_HMI_Popup_StatusNum3/1 -> Bus Creator23/26  "OMAPve_y_HMI_Popup_Status_2"
  OMAPve_y_Vehicle_Lane_DisplayNum4/1 -> Bus Creator23/27  "OMAPve_y_Vehicle_Lane_Display_2"
  OMAPve_y_ACC_HMI_TgtDisp_FlagNum5/1 -> Bus Creator23/21  "OMAPve_y_ACC_HMI_TgtDisp_Flag_2"
  Data Type Conversion29/1 -> Bus Creator14/3  "OMAPve_g_Coefficient_toregulate_EPS_2"
  OMAPve_y_Hands_off_warningNum3/1 -> Bus Creator23/25  "OMAPve_y_Hands_off_warning_2"
  OMAPve_y_LKA_action_indicationNum3/1 -> Bus Creator23/33  "OMAPve_y_LKA_action_indication_2"
  OMAPve_y_LKA_Mode_from_CameraNum4/1 -> Bus Creator23/30  "OMAPve_y_LKA_Mode_from_Camera_2"
  Constant1/1 -> Bus Creator14/2  "OMAPve_y_General_state_of_LKA_function3F2_2"
  OMAPve_y_RVVACC_Vehiclespeed_request_typeNum5/1 -> Bus Creator23/14  "OMAPve_y_RVVACC_Vehiclespeed_request_type_2"
  Data Type Conversion31/1 -> Bus Creator14/5  "OMAPve_y_Permit_to_know_if_LKA_or_LPA3F2_2"
  OMAPve_y_LDW_FlagNum4/1 -> Bus Creator23/28  "OMAPve_y_LDW_Flag_2"
  Constant23/1 -> Bus Creator14/1  "OMAPve_y_Power_steering_power_cut3F2_2"
  OMAPve_y_ACC_DesiredHeadway_Icon_BasicNum5/1 -> Bus Creator23/10  "OMAPve_y_ACC_DesiredHeadway_Icon_Basic_2"
  OMAPve_y_State_of_the_functionFARC_detNum/1 -> Bus Creator5/2  "OMAPve_y_State_of_the_functionFARC_det_1"
  OMAPve_y_Haptic_AlarmNum/1 -> Bus Creator5/5  "OMAPve_y_Haptic_Alarm_1"
  OMAPve_y_FCW_StatusNum/1 -> Bus Creator5/1  "OMAPve_y_FCW_Status_1"
  OMAPve_y_MDD_deceleration_typeNum/1 -> Bus Creator5/10  "OMAPve_y_MDD_deceleration_type_1"
  Bus Creator5/1 -> ESA_ESC/1  "ESA_ESC"
  OMAPve_y_MDD_Decelerationcontrol_requestNum/1 -> Bus Creator5/9  "OMAPve_y_MDD_Decelerationcontrol_request_1"
  OMAPve_y_AEB_Braking_progressNum/1 -> Bus Creator5/12  "OMAPve_y_AEB_Braking_progress_1"
  OMAPve_y_AEB_StatusNum/1 -> Bus Creator5/3  "OMAPve_y_AEB_Status_1"
  OMAPve_g_Deceleration_setpoint_deviceNum/1 -> Bus Creator5/8  "OMAPve_g_Deceleration_setpoint_device_1"
  OMAPve_g_ACCTqReqNum/1 -> Bus Creator/3  "OMAPve_g_ACCTqReq_1"
  Bus Creator/1 -> ESA_EMS/1  "ESA_EMS"
  OMAPve_g_PotACCTqReqNum/1 -> Bus Creator/2  "OMAPve_g_PotACCTqReq_1"
  OMAPve_y_ACC_Engine_Start_RequestNum/1 -> Bus Creator/1  "OMAPve_y_ACC_Engine_Start_Request_1"
  OMAPve_y_stAcvTqWhlPTPotReqNum/1 -> Bus Creator/6  "OMAPve_y_stAcvTqWhlPTPotReq_1"
  OMAPve_y_Decel_RequestNum/1 -> Bus Creator5/11  "OMAPve_y_Decel_Request_1"
  OMAPve_y_Function_Acc_statusNum/1 -> Bus Creator/7  "OMAPve_y_Function_Acc_status_1"
  OMAPve_g_TminUp_or_downGearNum/1 -> Bus Creator/5  "OMAPve_g_TminUp_or_downGear_1"
  OMAPve_y_Prefill_requestNum/1 -> Bus Creator5/4  "OMAPve_y_Prefill_request_1"
  OMAPve_y_Powertrain_torquewheel_requestNum/1 -> Bus Creator/4  "OMAPve_y_Powertrain_torquewheel_request_1"
  Input_FDMM/1 -> Terminator1/1
  OMAPve_y_ADAS_ELKStsNum1/1 -> Bus Creator23/34  "OMAPve_y_ADAS_ELKSts_2"
  OMAPve_y_ADAS_ESCHoldReqNum/1 -> Bus Creator5/7  "OMAPve_y_ADAS_ESCHoldReq"
  OMAPve_y_ADAS_ESCDriveOffNum/1 -> Bus Creator5/6  "OMAPve_y_ADAS_ESCDriveOff"
  OMAPve_y_ADAS_ACCRequestEPBNum/1 -> Bus Creator5/13  "OMAPve_y_ADAS_ACCRequestEPB"
  OMAPve_y_ADAS_JAFaultSt_2/1 -> Bus Creator23/20  "OMAPve_y_ADAS_JAFaultSt_2"
  OMAPve_y_ADAS_ISLCState1/1 -> Bus Creator23/23  "OMAPve_y_ADAS_ISLCState_2"
  OMAPve_y_ADAS_ISLCDriverRemind1/1 -> Bus Creator23/24  "OMAPve_y_ADAS_ISLCDriverRemind_2"
  OMAPve_y_ADAS_HWAActionSts/1 -> Bus Creator23/4  "OMAPve_y_ADAS_HWAActionSts_2"
  OMAPve_y_ADAS_HWAMode/1 -> Bus Creator23/7  "OMAPve_y_ADAS_HWAMode_2"
  OMAPve_y_ADAS_TurnLightsCommand1/1 -> Bus Creator23/5  "OMAPve_y_ADAS_TurnLightsCommand_2"
  OMAPve_y_ADAS_HWATurnOnIndicator/1 -> Bus Creator23/3  "OMAPve_y_ADAS_HWATurnOnIndicator_2"
  OMAPve_y_ADAS_LightControlValid/1 -> Bus Creator23/6  "OMAPve_y_ADAS_LightControlValid_2"
  Input_ESAS/1 -> Bus Selector1/1, Bus Selector/1
  Bus Selector/1 -> Data Type Conversion29/1  "<ESASve_g_EPS_Factor_Control_convert>"
  Bus Selector/2 -> Data Type Conversion30/1  "<ESASve_g_ESA_SWA_CMD_convert>"
  Bus Selector/3 -> Data Type Conversion31/1  "<ESASve_y_LKAActivation_convert>"
  Bus Selector/4 -> Data Type Conversion1/1  "<ESASve_y_ESA_State_convert>"
  Data Type Conversion1/1 -> Bus Creator14/6  "OMAPve_y_ADAS_ESAState_2"
  Bus Selector/6 -> Data Type Conversion2/1  "<ESASve_y_ESARequest_convert>"
  Data Type Conversion2/1 -> Bus Creator14/8  "OMAPve_y_ADAS_ESARequest_2"
  Bus Selector/5 -> Data Type Conversion3/1  "<ESASve_y_ESATorqueReq_convert>"
  Data Type Conversion3/1 -> Bus Creator14/7  "OMAPve_g_ADAS_ESATorqueReq_2"
  Data Type Conversion4/1 -> Bus Creator23/2  "OMAPve_y_ADAS_ESAFaultSt_2"
  Bus Selector1/1 -> Data Type Conversion4/1  "<ESASve_y_ESA_FaultSt_convert>"
  Constant4/1 -> Bus Creator23/1  "OMAPve_y_ADAS_ELKPopupMessage_2"

== system OMAP/Runnable_OMAP_10ms_sys/OMAP_Module/ICA_Direct_G59 ==
  note: 配OMAP_G59
  note: 修改内容：G59 ET0车上与EPS的握手信号
      | 24 :增加转向灯命令信号，并为此信号增加两个标定量
      | 25:首次适配G59HMI，将车道线显示、文字显示、图标显示、声音提示均进行了适配修改，同时新增变道功能相关输出信号OMAPve_y_ADAS_HWATurnOnIndicator_2（请驾驶员拨转向杆确认变道）、OMAPve_y_ADAS_HWAActionSts_2（显示正在往左或是往右变道画面）、OMAPve_y_ADAS_LightControlValid_2（ADAS控转向灯有效性）、OMAPve_y_ADAS_TurnLightsCommand_2（ADAS控转向灯信号）、OMAPve_y_ADAS_HWAMode_2（多车道模式图标信号）。
      | 参考文档：OMAP接口文档3.6、HMI显示需求1.4、信号矩阵V2.1
      | 匹配模型：OMAP_ver032
      | 26:LKA activation控车与否都输出0
      | 27：取消降级达到恢复超时后橙色闪烁的设计，接入ICA模式开关信号、变道打转向灯信号，为HWATurnOnIndicator接入内容
      | 28：驾驶员立即接管触发条件新增车辆非静止
      | 29：经与G35商议一致，取消进入降级时的警示音（handsoffwarning）；把运算中的TH_MODE换为TH_STATE；增加标定量Clb_ICADirect_TrnLghtsCrtl_Inhb指示是否禁止控转向灯
      | 30:当ACC切ICA时，亮黄灯；从头开始开启ICA时，保持亮灰灯
      | 31：把上次改过的ICA icon这一块做了标定量，方便以后调试
      | 32:根据实车测试结果，实施ICA_ICON的更改，优化ACC切ICA时的HMI连续性; 根据对G35等竞品调研，增加扭矩系数变化率相关标定量
      | 33：修改车道线显示模块，显示方式设置两种，简单的只显示双灰双蓝，或者可显示单侧车道线，调试后确定一种；增加显示数值标定量。
  Input_ICA : Inport
  Input_FDMM : Inport  Port=2
  Input_IMAP : Inport  Port=3
  ACC_to_ICA : Inport  Port=4
  Bus Creator : BusCreator  Inputs=2
  Bus Creator15 : BusCreator  Inputs=8
  Bus Creator24 : BusCreator  Inputs=36
  Bus Selector : BusSelector  OutputSignals=OMAPve_y_General_state_of_LKA_function3F2_2,OMAPve_g_Coefficient_toregulate_EPS_2,ICABve_g_SteerAngleCmd_convert,OMAPve_y_Permit_to_know_if_LKA_or_LPA3F2_2,ICABve_d_LKATorqueReq_convert,ICABve_g_LKATorqueReq_Value_convert
  Bus Selector1 : BusSelector  OutputSignals=OMAPve_y_ADAS_HWATurnOnIndicator_2,OMAPve_y_ADAS_HWAActionSts_2,OMAPve_y_ADAS_TurnLightsCommand_2,OMAPve_y_ADAS_LightControlValid_2,OMAPve_y_ADAS_HWAMode_2,OMAPve_y_TSR_Vision_Only_Sign_Type_2,OMAPve_y_ISA_Value_2,OMAPve_y_Hands_off_warning_2,OMAPve_y_Vehicle_Lane_Display_2,OMAPve_y_ICA_HMI_Txt_Disp_2,OMAPve_y_TJA_status_icon_2
  Bus Selector2 : BusSelector  OutputSignals=OMAPve_y_ACC_DesiredHeadway_Display_2,OMAPve_y_ACC_DesiredHeadway_Icon_Basic_2,OMAPve_y_ACC_Desired_Set_Speed_2,OMAPve_y_ACC_Set_Speed_Display_2,OMAPve_y_ACC_Vehicle_Icon_Display_2,OMAPve_y_RVVACC_Vehiclespeed_request_type_2,ACCSve_d_ACCMessagePrompt_convert,OMAPve_y_ACC_HMI_TgtDisp_Flag_2,OMAPve_y_TARGET_POSITION_2,ACCSve_d_ACC_ISLCState_convert,ACCSve_d_ACC_ISLCDriverRemind_convert
  Constant{,2..4} (4 alike) : Constant  Value=0  OutDataTypeStr=uint8
  Constant1 : Constant  Value=0  OutDataTypeStr=single
  Constant27 : Constant  Value=33  OutDataTypeStr=uint16
  Data Type Conversion1 : DataTypeConversion  OutDataTypeStr=single
  Data Type Conversion{3..5,7..20,22..25,28,46..47} (24 alike) : DataTypeConversion  OutDataTypeStr=uint8
  Data Type Conversion2 : DataTypeConversion  OutDataTypeStr=single
  Data Type Conversion21 : DataTypeConversion  OutDataTypeStr=single
  ICA_Define : Subsystem
  OMAPve_y_ADAS_ELKStsNum1 : Constant  Value=0  OutDataTypeStr=uint8
  OMAPve_y_ADAS_JAFaultSt_2 : Constant  Value=0  OutDataTypeStr=uint8
  OMAPve_y_AEB_Alert_ReqNum4 : Constant  Value=0  OutDataTypeStr=uint8
  OMAPve_y_AEB_Fault_StatusNum4 : Constant  Value=0  OutDataTypeStr=uint8
  OMAPve_y_AEB_Switch_StatusNum4 : Constant  Value=0  OutDataTypeStr=uint8
  OMAPve_y_AEB_tipsNum4 : Constant  Value=0  OutDataTypeStr=uint8
  OMAPve_y_HMI_Popup_StatusNum4 : Constant  Value=0  OutDataTypeStr=uint8
  OMAPve_y_LDW_FlagNum5 : Constant  Value=0  OutDataTypeStr=uint8
  OMAPve_y_LDW_Status_DisplayNum5 : Constant  Value=0  OutDataTypeStr=uint8
  OMAPve_y_LKA_Mode_from_CameraNum5 : Constant  Value=0  OutDataTypeStr=uint8
  OMAPve_y_LKA_Status_DisplayNum4 : Constant  Value=0  OutDataTypeStr=uint8
  OMAPve_y_LKA_Switch_StateNum5 : Constant  Value=0  OutDataTypeStr=uint8
  OMAPve_y_LKA_action_indicationNum4 : Constant  Value=0  OutDataTypeStr=uint8
  OMAPve_y_Power_steering_power_cut3F2Num2 : Constant  Value=0  OutDataTypeStr=uint8
  Terminator : Terminator
  Terminator1 : Terminator
  Terminator2 : Terminator
  ICA_EPS : Outport
  ICA_IC : Outport  Port=2
  ICA_Input : Outport  Port=3
  wires:
  OMAPve_y_AEB_Alert_ReqNum4/1 -> Bus Creator24/16  "OMAPve_y_AEB_Alert_Req_2"
  Data Type Conversion16/1 -> Bus Creator24/14  "OMAPve_y_RVVACC_Vehiclespeed_request_type_2"
  Bus Selector1/8 -> Data Type Conversion7/1  "<OMAPve_y_Hands_off_warning_2>"
  Data Type Conversion12/1 -> Bus Creator24/10  "OMAPve_y_ACC_DesiredHeadway_Icon_Basic_2"
  Bus Selector1/7 -> ?  "<OMAPve_y_ISA_Value_2>"
  Data Type Conversion14/1 -> Bus Creator24/12  "OMAPve_y_ACC_Set_Speed_Display_2"
  OMAPve_y_LDW_FlagNum5/1 -> Bus Creator24/28  "OMAPve_y_LDW_Flag_2"
  Bus Creator24/1 -> ICA_IC/1  "ICA_IC"
  OMAPve_y_AEB_tipsNum4/1 -> Bus Creator24/19  "OMAPve_y_AEB_tips_2"
  Bus Selector1/11 -> Data Type Conversion9/1  "<OMAPve_y_TJA_status_icon_2>"
  Data Type Conversion13/1 -> Bus Creator24/11  "OMAPve_y_ACC_Desired_Set_Speed_2"
  OMAPve_y_LKA_Status_DisplayNum4/1 -> Bus Creator24/31  "OMAPve_y_LKA_Status_Display_2"
  Data Type Conversion18/1 -> Bus Creator24/21  "OMAPve_y_ACC_HMI_TgtDisp_Flag_2"
  Data Type Conversion17/1 -> Bus Creator24/15  "OMAPve_y_ACC_Pop_Up_Message_2"
  OMAPve_y_LKA_Switch_StateNum5/1 -> Bus Creator24/32  "OMAPve_y_LKA_Switch_State_2"
  Data Type Conversion15/1 -> Bus Creator24/13  "OMAPve_y_ACC_Vehicle_Icon_Display_2"
  Bus Selector1/10 -> Data Type Conversion10/1  "<OMAPve_y_ICA_HMI_Txt_Disp_2>"
  OMAPve_y_LKA_Mode_from_CameraNum5/1 -> Bus Creator24/30  "OMAPve_y_LKA_Mode_from_Camera_2"
  OMAPve_y_LDW_Status_DisplayNum5/1 -> Bus Creator24/29  "OMAPve_y_LDW_Status_Display_2"
  OMAPve_y_AEB_Fault_StatusNum4/1 -> Bus Creator24/17  "OMAPve_y_AEB_Fault_Status_2"
  Bus Selector1/6 -> Data Type Conversion4/1  "<OMAPve_y_TSR_Vision_Only_Sign_Type_2>"
  OMAPve_y_HMI_Popup_StatusNum4/1 -> Bus Creator24/26  "OMAPve_y_HMI_Popup_Status_2"
  Bus Creator15/1 -> ICA_EPS/1  "ICA_EPS"
  Data Type Conversion11/1 -> Bus Creator24/9  "OMAPve_y_ACC_DesiredHeadway_Display_2"
  Data Type Conversion19/1 -> Bus Creator24/22  "OMAPve_y_TARGET_POSITION_2"
  OMAPve_y_AEB_Switch_StatusNum4/1 -> Bus Creator24/18  "OMAPve_y_AEB_Switch_Status_2"
  OMAPve_y_LKA_action_indicationNum4/1 -> Bus Creator24/33  "OMAPve_y_LKA_action_indication_2"
  Bus Selector1/9 -> Data Type Conversion8/1  "<OMAPve_y_Vehicle_Lane_Display_2>"
  Input_ICA/1 -> ICA_Define/1(In1)
  Input_IMAP/1 -> ICA_Define/3(In2)
  Input_FDMM/1 -> ICA_Define/2(In3)
  ACC_to_ICA/1 -> Bus Selector2/1, ICA_Define/4(In4)
  ICA_Define/2(Out2) -> Bus Creator/2, Bus Selector1/1  "HMI"
  Bus Creator/1 -> ICA_Input/1
  Data Type Conversion4/1 -> Bus Creator24/8  "OMAPve_y_TSR_Vision_Only_Sign_Type_2"
  Data Type Conversion7/1 -> Bus Creator24/25  "OMAPve_y_Hands_off_warning_2"
  Data Type Conversion8/1 -> Bus Creator24/27  "OMAPve_y_Vehicle_Lane_Display_2"
  Data Type Conversion9/1 -> Bus Creator24/36  "OMAPve_y_TJA_status_icon_2"
  Data Type Conversion10/1 -> Bus Creator24/35  "OMAPve_y_ICA_HMI_Txt_Disp_2"
  Bus Selector2/1 -> Data Type Conversion11/1  "<OMAPve_y_ACC_DesiredHeadway_Display_2>"
  Bus Selector2/2 -> Data Type Conversion12/1  "<OMAPve_y_ACC_DesiredHeadway_Icon_Basic_2>"
  Bus Selector2/3 -> Data Type Conversion13/1  "<OMAPve_y_ACC_Desired_Set_Speed_2>"
  Bus Selector2/4 -> Data Type Conversion14/1  "<OMAPve_y_ACC_Set_Speed_Display_2>"
  Bus Selector2/5 -> Data Type Conversion15/1  "<OMAPve_y_ACC_Vehicle_Icon_Display_2>"
  Bus Selector2/6 -> Data Type Conversion16/1  "<OMAPve_y_RVVACC_Vehiclespeed_request_type_2>"
  Bus Selector2/7 -> Data Type Conversion17/1  "<ACCSve_d_ACCMessagePrompt_convert>"
  Bus Selector2/8 -> Data Type Conversion18/1  "<OMAPve_y_ACC_HMI_TgtDisp_Flag_2>"
  Bus Selector2/9 -> Data Type Conversion19/1  "<OMAPve_y_TARGET_POSITION_2>"
  OMAPve_y_ADAS_ELKStsNum1/1 -> Bus Creator24/34  "OMAPve_y_ADAS_ELKSts_2"
  Data Type Conversion3/1 -> Bus Creator15/5  "OMAPve_y_Permit_to_know_if_LKA_or_LPA3F2_2"
  Bus Selector/5 -> Data Type Conversion20/1  "<ICABve_d_LKATorqueReq_convert>"
  Bus Selector/1 -> Data Type Conversion28/1  "<OMAPve_y_General_state_of_LKA_function3F2_2>"
  Bus Selector/4 -> Data Type Conversion3/1  "<OMAPve_y_Permit_to_know_if_LKA_or_LPA3F2_2>"
  Bus Selector/6 -> Data Type Conversion21/1  "<ICABve_g_LKATorqueReq_Value_convert>"
  Data Type Conversion20/1 -> Terminator/1  "OMAPve_y_DAS4_Status_LKATorqueReq"
  Bus Selector/2 -> Data Type Conversion1/1  "<OMAPve_g_Coefficient_toregulate_EPS_2>"
  OMAPve_y_Power_steering_power_cut3F2Num2/1 -> Bus Creator15/1  "OMAPve_y_Power_steering_power_cut3F2_2"
  Data Type Conversion1/1 -> Bus Creator15/3  "OMAPve_g_Coefficient_toregulate_EPS_2"
  Data Type Conversion28/1 -> Bus Creator15/2  "OMAPve_y_General_state_of_LKA_function3F2_2"
  Data Type Conversion21/1 -> Terminator1/1  "OMAPve_g_DAS4_Status_LKATorqueReq_Value"
  ICA_Define/1(Out1) -> Bus Selector/1, Bus Creator/1  "actuator"
  Bus Selector/3 -> Data Type Conversion2/1  "<ICABve_g_SteerAngleCmd_convert>"
  Data Type Conversion2/1 -> Bus Creator15/4  "OMAPve_g_Column_angle_setpoint3F2_2"
  Constant27/1 -> Terminator2/1  "ob_OMAP_ICAdirect_version"
  OMAPve_y_ADAS_JAFaultSt_2/1 -> Bus Creator24/20  "OMAPve_y_ADAS_JAFaultSt_2"
  Bus Selector1/3 -> Data Type Conversion5/1  "<OMAPve_y_ADAS_TurnLightsCommand_2>"
  Data Type Conversion5/1 -> Bus Creator24/5  "OMAPve_y_ADAS_TurnLightsCommand_2"
  Bus Selector1/1 -> Data Type Conversion22/1  "<OMAPve_y_ADAS_HWATurnOnIndicator_2>"
  Data Type Conversion22/1 -> Bus Creator24/3  "OMAPve_y_ADAS_HWATurnOnIndicator_2"
  Data Type Conversion23/1 -> Bus Creator24/4  "OMAPve_y_ADAS_HWAActionSts_2"
  Bus Selector1/2 -> Data Type Conversion23/1  "<OMAPve_y_ADAS_HWAActionSts_2>"
  Data Type Conversion24/1 -> Bus Creator24/6  "OMAPve_y_ADAS_LightControlValid_2"
  Bus Selector1/4 -> Data Type Conversion24/1  "<OMAPve_y_ADAS_LightControlValid_2>"
  Bus Selector1/5 -> Data Type Conversion25/1  "<OMAPve_y_ADAS_HWAMode_2>"
  Data Type Conversion25/1 -> Bus Creator24/7  "OMAPve_y_ADAS_HWAMode_2"
  Data Type Conversion47/1 -> Bus Creator24/24  "OMAPve_y_ADAS_ISLCDriverRemind_2"
  Data Type Conversion46/1 -> Bus Creator24/23  "OMAPve_y_ADAS_ISLCState_2"
  Bus Selector2/10 -> Data Type Conversion46/1  "<ACCSve_d_ACC_ISLCState_convert>"
  Bus Selector2/11 -> Data Type Conversion47/1  "<ACCSve_d_ACC_ISLCDriverRemind_convert>"
  Constant1/1 -> Bus Creator15/7  "OMAPve_g_ADAS_ESATorqueReq_2"
  Constant/1 -> Bus Creator15/6  "OMAPve_y_ADAS_ESAState_2"
  Constant2/1 -> Bus Creator15/8  "OMAPve_y_ADAS_ESARequest_2"
  Constant3/1 -> Bus Creator24/2  "OMAPve_y_ADAS_ESAFaultSt_2"
  Constant4/1 -> Bus Creator24/1  "OMAPve_y_ADAS_ELKPopupMessage_2"
